simulink model "Q2"  (Simulink 7.6)
settings: Solver=ode45  StartTime=0.0  StopTime=10  MinStep=0.01  RelTol=1e-3
settings Model: Creator=AG65800  LastModifiedBy=AG65800

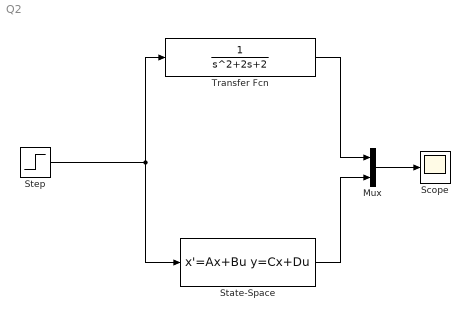
== system Q2 ==
  Mux : Mux  Inputs=2
  Scope : Scope
      settings: SaveName=y1  DataFormat=Array  SampleTime=0.1
  State-Space : StateSpace  A=[0 1; -2 -2 ]  B=[ 0 ; 1]  C="[1  0 ]"  D=[0]
  Step : Step  Time=0  SampleTime=0
  Transfer Fcn : TransferFcn  Denominator=[1 2 2]
  wires:
  Step/1 -> Transfer Fcn/1, State-Space/1
  Transfer Fcn/1 -> Mux/1
  State-Space/1 -> Mux/2
  Mux/1 -> Scope/1
